simulink model "zadatak2"  (R2017b)
settings: Solver=VariableStepAuto  StartTime=0.0  StopTime=600.0  RelTol=1e-3
undefined symbols (not defined in the file or in its folder): ln
libraries: simulink x4
settings Model: Creator=HP  LastModifiedBy=HP

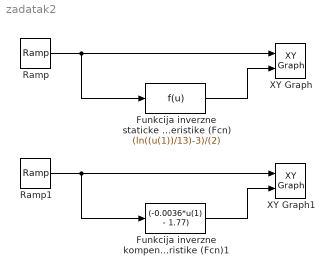
== system zadatak2 ==
  Funkcija inverzne kompenzirane karakteristike (Fcn)1 : Fcn  Expr=(-0.0036*u(1) - 1.77)
  Funkcija inverzne staticke karakteristike (Fcn) : Fcn  Expr=(ln((u(1))/13)-3)/(2)
  Ramp : simulink/Sources/Ramp  slope=1  start=0  X0=0
  Ramp1 : simulink/Sources/Ramp  slope=1  start=0  X0=0
  XY Graph : simulink/Sinks/XY Graph  xmin=-300  xmax=300  ymin=-1.5  ymax=0.068  st=1
  XY Graph1 : simulink/Sinks/XY Graph  xmin=-300  xmax=300  ymin=-2.85  ymax=-0.69  st=1
  wires:
  Funkcija inverzne staticke karakteristike (Fcn)/1 -> XY Graph/2
  Ramp/1 -> Funkcija inverzne staticke karakteristike (Fcn)/1, XY Graph/1
  Ramp1/1 -> Funkcija inverzne kompenzirane karakteristike (Fcn)1/1, XY Graph1/1
  Funkcija inverzne kompenzirane karakteristike (Fcn)1/1 -> XY Graph1/2
